simulink model "Aproximado"  (Simulink 5.0)
settings: Solver=ode45  StartTime=0.0  StopTime=100.0  RelTol=1e-3
undefined symbols (not defined in the file): ts
libraries: dspmtrx3 x6, simulink x4
settings Model: LastModifiedBy=LeO

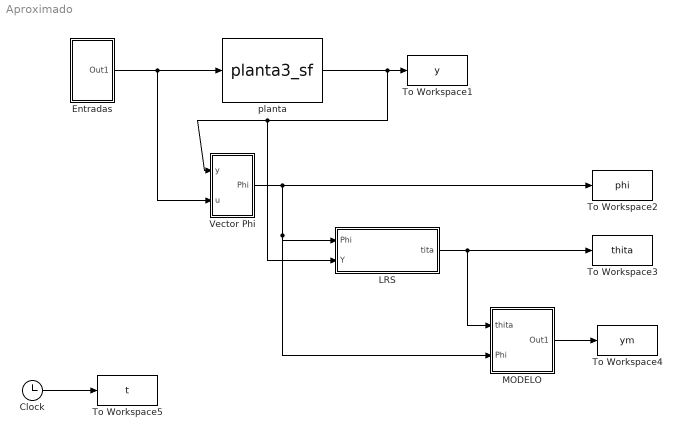
== system Aproximado ==
  Clock : Clock
      settings: Decimation=10
  Entradas : Subsystem
  LRS : Subsystem  mask{mu=0.5}
      mask prompts: mu "factor de convergencia (mu)"
  MODELO : Subsystem
  To Workspace1 : ToWorkspace  VariableName=y  SampleTime=ts  SaveFormat=Array
  To Workspace2 : ToWorkspace  VariableName=phi  SampleTime=ts  SaveFormat=Array
  To Workspace3 : ToWorkspace  VariableName=thita  SampleTime=ts  SaveFormat=Array
  To Workspace4 : ToWorkspace  VariableName=ym  SampleTime=ts  SaveFormat=Array
  To Workspace5 : ToWorkspace  VariableName=t  SampleTime=ts  SaveFormat=Array
  Vector Phi : Subsystem  mask{nu=1, ny=3, nk=1}
      mask prompts: nu "Nº de u tomadas"; ny "Nº de y tomadas"; nk "Nº de retardo"
  planta : S-Function  FunctionName=planta3_sf
  wires:
  Entradas/1(Out1) -> Vector Phi/2(u), planta/1
  planta/1 -> To Workspace1/1, Vector Phi/1("y "), LRS/2(Y)
  Vector Phi/1(Phi) -> To Workspace2/1, LRS/1("Phi "), MODELO/2(Phi)
  Clock/1 -> To Workspace5/1
  LRS/1(tita) -> To Workspace3/1, MODELO/1(thita)
  MODELO/1(Out1) -> To Workspace4/1

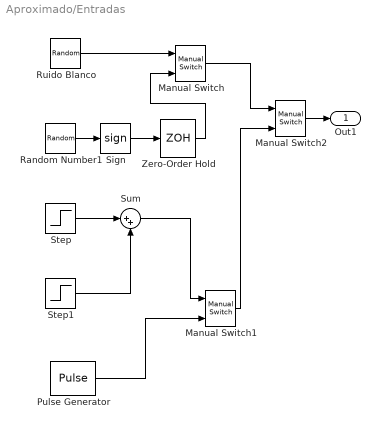
== system Aproximado/Entradas ==
  Manual Switch : simulink/Signal Routing/Manual Switch  sw=0  action=0
  Manual Switch1 : simulink/Signal Routing/Manual Switch  sw=1  action=0
  Manual Switch2 : simulink/Signal Routing/Manual Switch  sw=0  action=0
  Pulse Generator : DiscretePulseGenerator  PulseType=Time based  PulseWidth=50
  Random Number1 : RandomNumber  SampleTime=0
  Ruido Blanco : RandomNumber  Variance=20  Seed=12  SampleTime=ts
  Sign : Signum
  Step : Step  Time=10  After=25  SampleTime=0.05
  Step1 : Step  Time=30  After=3  SampleTime=0.05
  Sum : Sum  Inputs=|++  SaturateOnIntegerOverflow=on
  Zero-Order Hold : ZeroOrderHold  SampleTime=0.05
  Out1 : Outport
  wires:
  Sign/1 -> Zero-Order Hold/1
  Random Number1/1 -> Sign/1
  Manual Switch/1 -> Manual Switch2/1
  Ruido Blanco/1 -> Manual Switch/1
  Zero-Order Hold/1 -> Manual Switch/2
  Manual Switch2/1 -> Out1/1
  Step/1 -> Sum/1
  Step1/1 -> Sum/2
  Manual Switch1/1 -> Manual Switch2/2
  Sum/1 -> Manual Switch1/1
  Pulse Generator/1 -> Manual Switch1/2

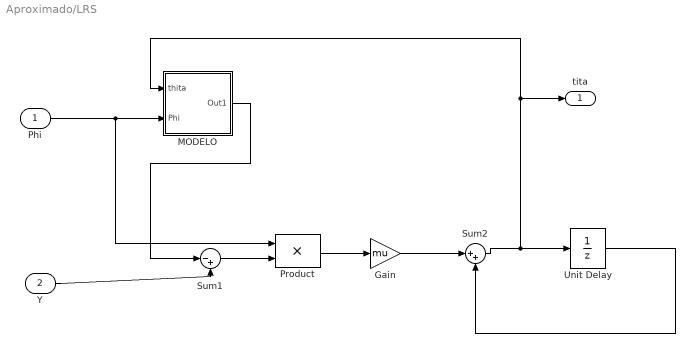
== system Aproximado/LRS ==
  "Phi " : Inport  SampleTime=ts
  Y : Inport  Port=2  SampleTime=ts
  Gain : Gain  Gain=mu  SaturateOnIntegerOverflow=on
  MODELO : Subsystem
  Product : Product  SaturateOnIntegerOverflow=on
  Sum1 : Sum  Inputs=|-+  SaturateOnIntegerOverflow=on
  Sum2 : Sum  Inputs=|++  SaturateOnIntegerOverflow=on
  Unit Delay : UnitDelay  X0=1*10^-3  SampleTime=ts
  tita : Outport
  wires:
  Unit Delay/1 -> Sum2/2
  "Phi "/1 -> MODELO/2(Phi), Product/1
  MODELO/1(Out1) -> Sum1/1
  Y/1 -> Sum1/2
  Product/1 -> Gain/1
  Gain/1 -> Sum2/1
  Sum2/1 -> Unit Delay/1, tita/1, MODELO/1(thita)
  Sum1/1 -> Product/2

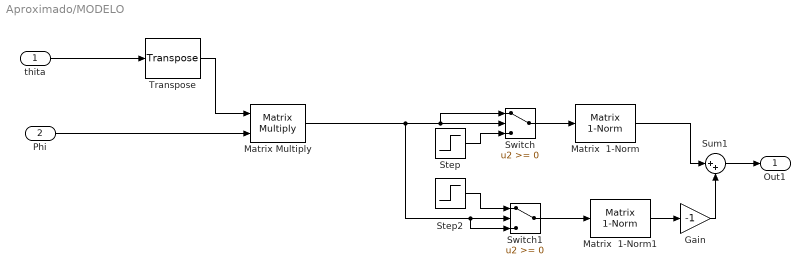
== system Aproximado/MODELO ==
  thita : Inport
  Phi : Inport  Port=2
  Gain : Gain  Gain=-1  SaturateOnIntegerOverflow=on
  Matrix  1-Norm : dspmtrx3/Matrix  1-Norm
  Matrix  1-Norm1 : dspmtrx3/Matrix  1-Norm
  Matrix Multiply : dspmtrx3/Matrix Multiply  numInputPorts=2  OptimizationLevel=None
  Step : Step  Time=0  After=0  SampleTime=0
  Step2 : Step  Time=0  After=0  SampleTime=0
  Sum1 : Sum  Inputs=|++  SaturateOnIntegerOverflow=on
  Switch : Switch  SaturateOnIntegerOverflow=on
  Switch1 : Switch  SaturateOnIntegerOverflow=on
  Transpose : dspmtrx3/Transpose  Hermitian=off
  Out1 : Outport
  wires:
  Phi/1 -> Matrix Multiply/2
  Transpose/1 -> Matrix Multiply/1
  thita/1 -> Transpose/1
  Matrix Multiply/1 -> Switch/2, Switch/1, Switch1/2, Switch1/3
  Sum1/1 -> Out1/1
  Step/1 -> Switch/3
  Switch/1 -> Matrix  1-Norm/1
  Switch1/1 -> Matrix  1-Norm1/1
  Step2/1 -> Switch1/1
  Matrix  1-Norm/1 -> Sum1/1
  Matrix  1-Norm1/1 -> Gain/1
  Gain/1 -> Sum1/2

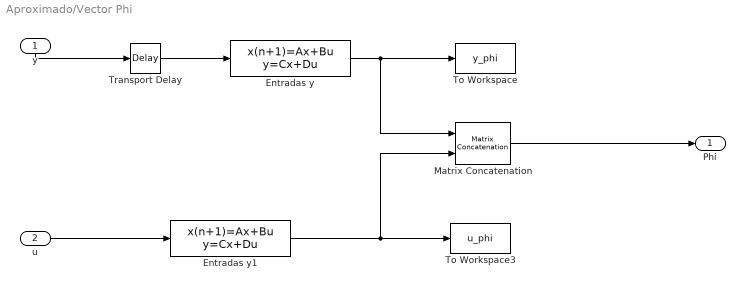
== system Aproximado/Vector Phi ==
  "y " : Inport  Orientation=down  SampleTime=ts
  u : Inport  Port=2  SampleTime=ts
  Entradas y : DiscreteStateSpace  A=[zeros(1,ny) ;eye(ny-1,ny)]  B=[[-1 zeros(1,ny-1)]']  C=[eye(ny)]  D=[zeros(1,ny)']  SampleTime=ts
  Entradas y1 : DiscreteStateSpace  A=[zeros(1,nu) ;eye(nu-1,nu)]  B=[[-1 zeros(1,nu-1)]']  C=[eye(nu)]  D=[zeros(1,nu)']  SampleTime=ts
  Matrix Concatenation : simulink/Math Operations/Matrix Concatenation  numInports=2  catMethod=Vertical
  To Workspace : ToWorkspace  VariableName=y_phi  SampleTime=ts  SaveFormat=Array
  To Workspace3 : ToWorkspace  VariableName=u_phi  SampleTime=ts  SaveFormat=Array
  Transport Delay : TransportDelay  DelayTime=nk*ts
  Phi : Outport
  wires:
  "y "/1 -> Transport Delay/1
  u/1 -> Entradas y1/1
  Entradas y/1 -> To Workspace/1, Matrix Concatenation/1
  Entradas y1/1 -> To Workspace3/1, Matrix Concatenation/2
  Matrix Concatenation/1 -> Phi/1
  Transport Delay/1 -> Entradas y/1

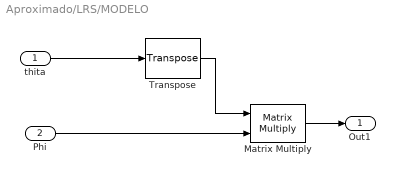
== system Aproximado/LRS/MODELO ==
  thita : Inport
  Phi : Inport  Port=2
  Matrix Multiply : dspmtrx3/Matrix Multiply  numInputPorts=2  OptimizationLevel=None
  Transpose : dspmtrx3/Transpose  Hermitian=off
  Out1 : Outport
  wires:
  Phi/1 -> Matrix Multiply/2
  Transpose/1 -> Matrix Multiply/1
  thita/1 -> Transpose/1
  Matrix Multiply/1 -> Out1/1
